simulink model "vi_du_2_str_r2015a"  (R2016b)
settings: Solver=ode4  StartTime=0.0  StopTime=100  FixedStep=0.1  RelTol=1e-3
undefined symbols (not defined in the file or in its folder): DiscIntNeverNeededParam
settings Model: Creator=ryell  LastModifiedBy=ADMIN
settings OptimizationCC: LifeSpan=inf
settings DebuggingCC: SFExecutionAtInitializationDiag=none
settings HardwareCC: ProdBitPerSizeT=32  ProdBitPerPtrDiffT=32  ProdWordSize=32  ProdHWDeviceType=Specified

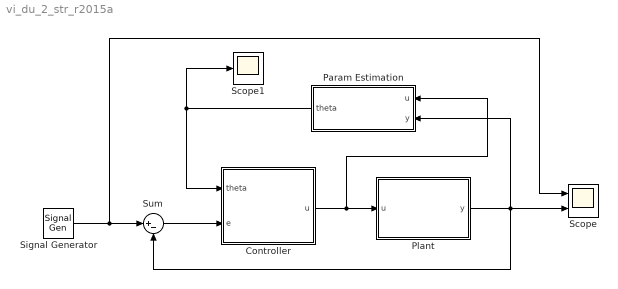
== system vi_du_2_str_r2015a ==
  Controller : Subsystem
  Param Estimation : Subsystem
  Plant : Subsystem
  Scope : Scope  NumInputPorts=2
  Scope1 : Scope
  Signal Generator : SignalGenerator  WaveForm=square  Frequency=0.1
  Sum : Sum  Inputs=|+-
  wires:
  Plant/1(y) -> Sum/2, Scope/2, Param Estimation/2(y)
  Controller/1(u) -> Param Estimation/1(u), Plant/1(u)
  Signal Generator/1 -> Scope/1, Sum/1
  Sum/1 -> Controller/2(e)
  Param Estimation/1(theta) -> Scope1/1, Controller/1(theta)

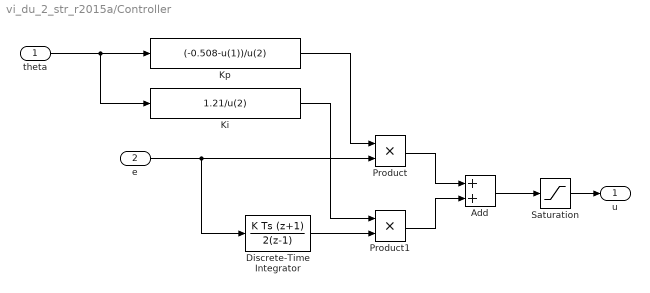
== system vi_du_2_str_r2015a/Controller ==
  theta : Inport
  e : Inport  Port=2
  Add : Sum
  Discrete-Time Integrator : DiscreteIntegrator  IntegratorMethod=Integration: Trapezoidal  InitialConditionSetting=State (most efficient)  SampleTime=-1  ICPrevOutput=DiscIntNeverNeededParam  ICPrevScaledInput=DiscIntNeverNeededParam
  Ki : Fcn  Expr=1.21/u(2)
  Kp : Fcn  Expr=(-0.508-u(1))/u(2)
  Product : Product
  Product1 : Product
  Saturation : Saturate  UpperLimit=10  LowerLimit=-10
  u : Outport
  wires:
  Discrete-Time Integrator/1 -> Product1/2
  e/1 -> Discrete-Time Integrator/1, Product/2
  Product/1 -> Add/1
  Product1/1 -> Add/2
  theta/1 -> Ki/1, Kp/1
  Kp/1 -> Product/1
  Ki/1 -> Product1/1
  Add/1 -> Saturation/1
  Saturation/1 -> u/1

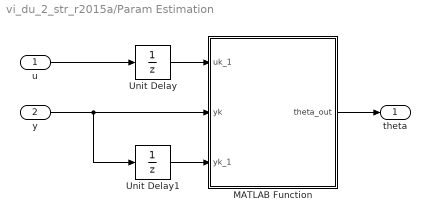
== system vi_du_2_str_r2015a/Param Estimation ==
  u : Inport
  y : Inport  Port=2
  MATLAB Function : MATLAB Function  TreatAsAtomicUnit=on
  Unit Delay : UnitDelay  SampleTime=-1
  Unit Delay1 : UnitDelay  SampleTime=-1
  theta : Outport
  wires:
  Unit Delay/1 -> MATLAB Function/1(uk_1)
  u/1 -> Unit Delay/1
  y/1 -> Unit Delay1/1, MATLAB Function/2(yk)
  Unit Delay1/1 -> MATLAB Function/3(yk_1)
  MATLAB Function/1(theta_out) -> theta/1

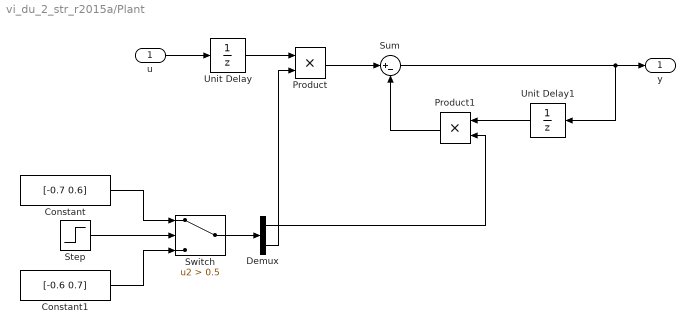
== system vi_du_2_str_r2015a/Plant ==
  u : Inport
  Constant : Constant  Value=[-0.7 0.6]
  Constant1 : Constant  Value=[-0.6 0.7]
  Demux : Demux  Outputs=2
  Product : Product
  Product1 : Product
  Step : Step  Time=50  SampleTime=0
  Sum : Sum  Inputs=|+-
  Switch : Switch  Criteria=u2 > Threshold  Threshold=0.5
  Unit Delay : UnitDelay  SampleTime=-1
  Unit Delay1 : UnitDelay  SampleTime=-1
  y : Outport
  wires:
  u/1 -> Unit Delay/1
  Unit Delay/1 -> Product/1
  Product/1 -> Sum/1
  Unit Delay1/1 -> Product1/1
  Product1/1 -> Sum/2
  Sum/1 -> Unit Delay1/1, y/1
  Step/1 -> Switch/2
  Constant/1 -> Switch/1
  Constant1/1 -> Switch/3
  Switch/1 -> Demux/1
  Demux/1 -> Product1/2
  Demux/2 -> Product/2

== matlab function vi_du_2_str_r2015a/Param Estimation/MATLAB Function ==
  data: uk_1 input; theta_out output; yk input; yk_1 input
function theta_out = fcn(uk_1,yk,yk_1)
persistent theta P

if (isempty(theta))
    theta = rand(2,1);
    P = 10*eye(2);
end

lambda = 0.95;

phi = [-yk_1;uk_1];

Lk = P*phi/(lambda + phi'*P*phi);
P = 1/lambda*(P-Lk*phi'*P);
ek = yk - phi'*theta;
theta = theta + Lk*ek;

theta_out = theta;
end
